simulink model "deneme_lineer_002"  (R2020b)
settings: Solver=VariableStepAuto  StartTime=0.0  StopTime=10.0  RelTol=1e-3
values from neighbouring files (symbols this model uses):
  u1max = 25*pi/180    (= 0.436332312999)    [RCAM_initialization.m]
  u1min = -25*pi/180    (= -0.436332312999)    [RCAM_initialization.m]
  u2max = 10*pi/180    (= 0.174532925199)    [RCAM_initialization.m]
  u2min = -25*pi/180    (= -0.436332312999)    [RCAM_initialization.m]
  u3max = 30*pi/180    (= 0.523598775598)    [RCAM_initialization.m]
  u3min = -30*pi/180    (= -0.523598775598)    [RCAM_initialization.m]
  u4max = 10*pi/180    (= 0.174532925199)    [RCAM_initialization.m]
  u4min = 0.5*pi/180    (= 0.00872664625997)    [RCAM_initialization.m]
  u5max = 10*pi/180    (= 0.174532925199)    [RCAM_initialization.m]
  u5min = 0.5*pi/180    (= 0.00872664625997)    [RCAM_initialization.m]
  x0 = [85; 0; 0; 0; 0; 0; 0; 0; 0; xini; yini; h0]    [RCAM_initialization.m]
undefined symbols (not defined in the file or in its folder): RCAM_MODEL_2
settings Model: Creator=Yigit  LastModifiedBy=Yigit

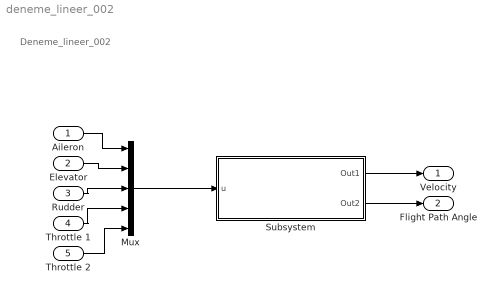
== system deneme_lineer_002 ==
  note: Deneme_lineer_002
  Aileron : Inport
  Elevator : Inport  Port=2
  Rudder : Inport  Port=3
  Throttle 1 : Inport  Port=4
  Throttle 2 : Inport  Port=5
  Mux : Mux  Inputs=5
  Subsystem : Subsystem
  Velocity : Outport
  Flight Path Angle : Outport  Port=2
  wires:
  Subsystem/2(Out2) -> Flight Path Angle/1
  Throttle 1/1 -> Mux/4
  Aileron/1 -> Mux/1
  Rudder/1 -> Mux/3
  Elevator/1 -> Mux/2
  Mux/1 -> Subsystem/1(u)
  Subsystem/1(Out1) -> Velocity/1
  Throttle 2/1 -> Mux/5

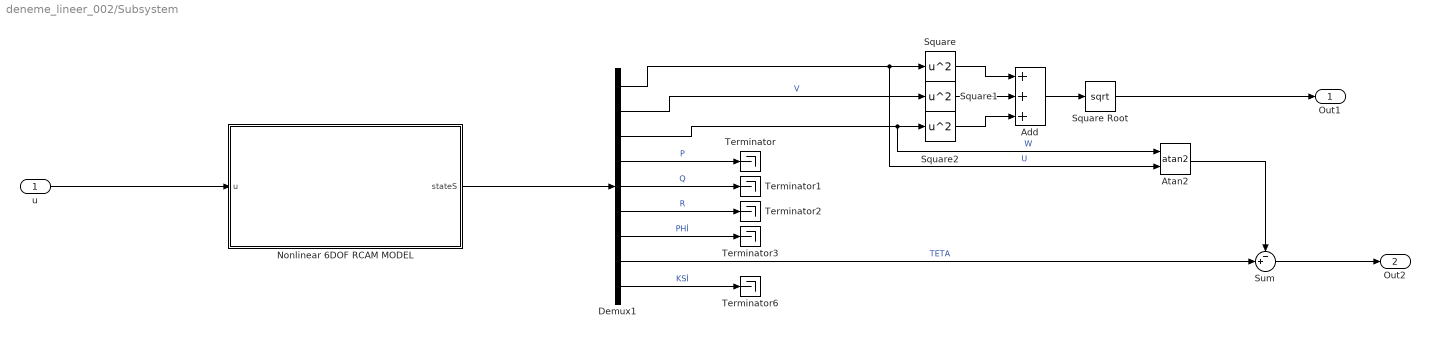
== system deneme_lineer_002/Subsystem ==
  u : Inport
  Add : Sum  Inputs=+++
  Atan2 : Trigonometry  Operator=atan2
  Demux1 : Demux  Outputs=9
  Nonlinear 6DOF RCAM MODEL : Subsystem
  Square : Math  Operator=square  SaturateOnIntegerOverflow=on
  Square Root : Sqrt  SaturateOnIntegerOverflow=on
  Square1 : Math  Operator=square  SaturateOnIntegerOverflow=on
  Square2 : Math  Operator=square  SaturateOnIntegerOverflow=on
  Sum : Sum  Inputs=-+|
  Terminator{,1..3,6} (5 alike) : Terminator
  Out1 : Outport
  Out2 : Outport  Port=2
  wires:
  Square2/1 -> Add/3
  Demux1/4 -> Terminator/1  "P"
  Add/1 -> Square Root/1
  Nonlinear 6DOF RCAM MODEL/1(stateS) -> Demux1/1
  Demux1/5 -> Terminator1/1  "Q"
  Demux1/1 -> Square/1, Atan2/2  "U"
  Demux1/3 -> Atan2/1, Square2/1  "W"
  Demux1/8 -> Sum/2  "TETA"
  Demux1/6 -> Terminator2/1  "R"
  Square Root/1 -> Out1/1
  Square/1 -> Add/1
  Demux1/9 -> Terminator6/1  "KSİ"
  Demux1/2 -> Square1/1  "V"
  Square1/1 -> Add/2
  u/1 -> Nonlinear 6DOF RCAM MODEL/1(u)
  Atan2/1 -> Sum/1
  Sum/1 -> Out2/1
  Demux1/7 -> Terminator3/1  "PHİ"

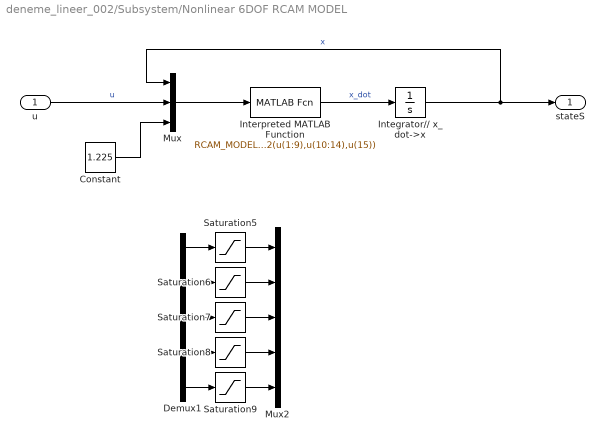
== system deneme_lineer_002/Subsystem/Nonlinear 6DOF RCAM MODEL ==
  u : Inport
  Constant : Constant  Value=1.225
  Demux1 : Demux  Outputs=5
  Integrator// x_dot->x : Integrator  InitialCondition=x0
  Interpreted MATLAB Function : MATLABFcn  MATLABFcn=RCAM_MODEL_2(u(1:9),u(10:14),u(15))
  Mux : Mux  Inputs=3
  Mux2 : Mux  Inputs=5
  Saturation5 : Saturate  UpperLimit=u1max  LowerLimit=u1min
  Saturation6 : Saturate  UpperLimit=u2max  LowerLimit=u2min
  Saturation7 : Saturate  UpperLimit=u3max  LowerLimit=u3min
  Saturation8 : Saturate  UpperLimit=u4max  LowerLimit=u4min
  Saturation9 : Saturate  UpperLimit=u5max  LowerLimit=u5min
  stateS : Outport
  wires:
  Interpreted MATLAB Function/1 -> Integrator// x_dot->x/1  "x_dot"
  Mux/1 -> Interpreted MATLAB Function/1
  Integrator// x_dot->x/1 -> stateS/1, Mux/1  "x"
  Constant/1 -> Mux/3
  Saturation6/1 -> Mux2/2
  Saturation8/1 -> Mux2/4
  Demux1/2 -> Saturation6/1
  Demux1/4 -> Saturation8/1
  Demux1/5 -> Saturation9/1
  Saturation7/1 -> Mux2/3
  Demux1/3 -> Saturation7/1
  Demux1/1 -> Saturation5/1
  Saturation5/1 -> Mux2/1
  Saturation9/1 -> Mux2/5
  u/1 -> Mux/2  "u"
